simulink model "example_of_minmax_block"  (R2021a)
settings: Solver=VariableStepAuto  StartTime=0.0  StopTime=10.0  MaxStep=1e-3  RelTol=1e-3
libraries: simulink x1
settings Model: Creator=YasserNet  LastModifiedBy=YasserNet

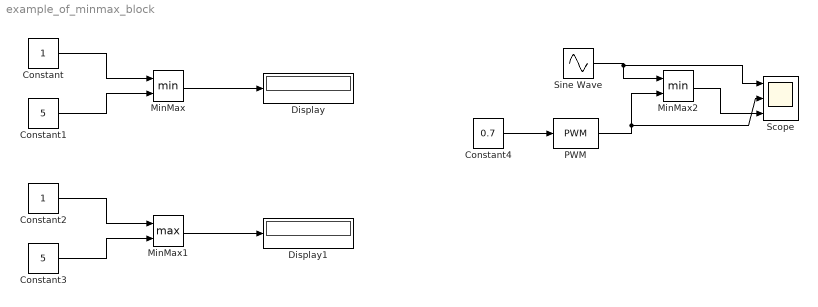
== system example_of_minmax_block ==
  Constant : Constant
  Constant1 : Constant  Value=5
  Constant2 : Constant
  Constant3 : Constant  Value=5
  Constant4 : Constant  Value=0.7
  Display : Display
  Display1 : Display
  MinMax : MinMax  Inputs=2
  MinMax1 : MinMax  Function=max  Inputs=2
  MinMax2 : MinMax  Inputs=2
  PWM : simulink/Discontinuities/PWM  DisableCoverage=on  Period=1  DisallowZeroDutyCycle=off  RunAtFixedTimeIntervals=off  SampleTime=0.1
  Scope : Scope  NumInputPorts=3
  Sine Wave : Sin  Frequency=2*2*pi  SampleTime=0
  wires:
  Constant/1 -> MinMax/1
  MinMax/1 -> Display/1
  Constant1/1 -> MinMax/2
  Constant3/1 -> MinMax1/2
  MinMax1/1 -> Display1/1
  Constant2/1 -> MinMax1/1
  Sine Wave/1 -> Scope/1, MinMax2/1
  PWM/1 -> Scope/2, MinMax2/2
  Constant4/1 -> PWM/1
  MinMax2/1 -> Scope/3
